simulink model "Model_pmsmdynamic"  (R2019b)
settings: Solver=ode4  StartTime=0.0  StopTime=2  RelTol=1e-3
InitFcn:
  | parameter
values from neighbouring files (symbols this model uses):
  b = 0.001    [parameter.m]
  f = 0.162    [parameter.m]
  j = 0.1    [parameter.m]
  kiid = 350    [parameter.m]
  kiiq = 350    [parameter.m]
  kis = 0.1    [parameter.m]
  kpid = 1.07    [parameter.m]
  kpiq = 1.07    [parameter.m]
  kps = 10    [parameter.m]
  Ld = 0.000538    [parameter.m]
  Lq = 0.000824    [parameter.m]
  p = 3    [parameter.m]
  rs = 0.0065    [parameter.m]
libraries: simulink x3
settings Model: ModifiedByFormat=Muhammad  Creator=Muhammad  LastModifiedBy=Muhammad
settings SolverCC: ZeroCrossAlgorithm=Adaptive
settings DataIOCC: ReturnWorkspaceOutputs=off
settings DebuggingCC: MaxConsecutiveZCsMsg=none  ArithmeticOperatorsInVariantConditions=warning
settings SFSimCC: SimUseLocalCustomCode=off  CustomCodeUndefinedFunction=UseInterfaceOnly
settings RTWCC: RTWUseLocalCustomCode=off

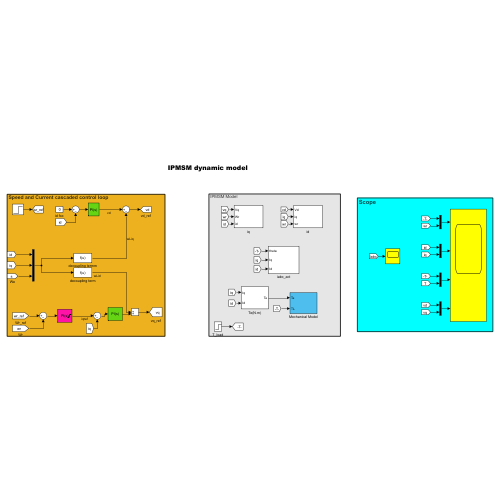
[thumbnail: Simulink's stored preview of the top-level diagram]
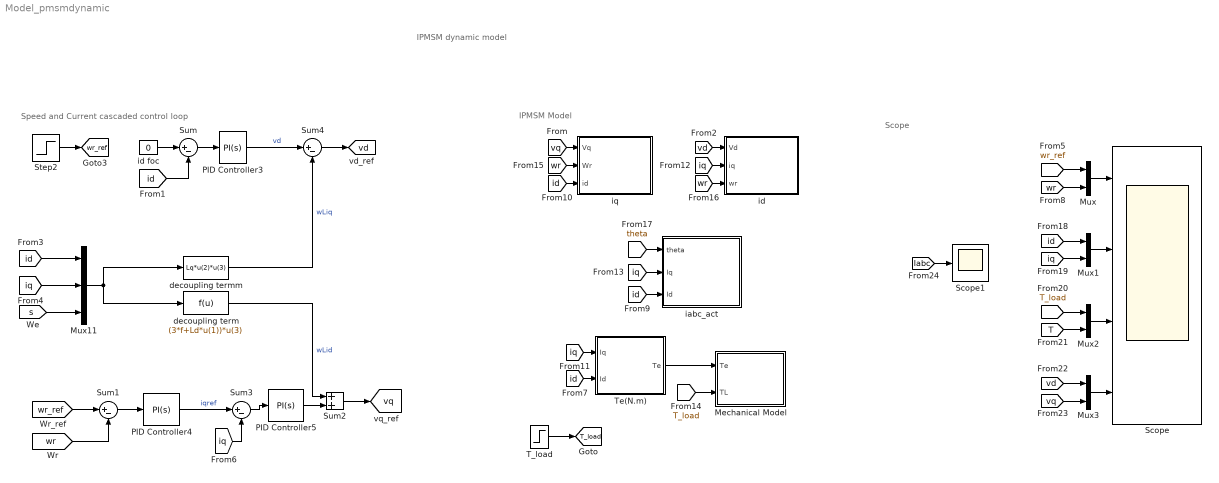
== system Model_pmsmdynamic ==
  note: Scope
  note: Speed and Current cascaded control loop
  note: IPMSM Model
  note: IPMSM dynamic model
  Mechanical Model : Subsystem
  Mux{,1..3} (4 alike) : Mux  Inputs=2
  Mux11 : Mux  Inputs=3
  PID Controller3 : simulink/Continuous/PID Controller  Controller=PI  Form=Parallel  TimeDomain=Continuous-time  SampleTime=0.0001  IntegratorMethod=Forward Euler  FilterMethod=Forward Euler  ControllerParametersSource=internal  P=kpid  I=kiid  D=0  N=100  UseFilter=on  TunerSelectOption=Transfer Function Based (PID Tuner App)  InitialConditionSource=internal  InitialConditionForIntegrator=0  InitialConditionForFilter=0  DifferentiatorICPrevScaledInput=0  ExternalReset=none  TrackingMode=off  Kt=1  LimitOutput=off  UpperSaturationLimit=800  LowerSaturationLimit=-800  LinearizeAsGain=on  AntiWindupMode=none  Kb=1  POutMin=[]  POutMax=[]  IOutMin=[]  IOutMax=[]  DOutMin=[]  DOutMax=[]  NOutMin=[]  NOutMax=[]  SumOutMin=[]  SumOutMax=[]  SaturationOutMin=[]  SaturationOutMax=[]  PParamMin=[]  PParamMax=[]  IParamMin=[]  IParamMax=[]  DParamMin=[]  DParamMax=[]  NParamMin=[]  NParamMax=[]  KbParamMin=[]  KbParamMax=[]  KtParamMin=[]  KtParamMax=[]  KbOutMin=[]  KbOutMax=[]  KtOutMin=[]  KtOutMax=[]  IntegratorOutMin=[]  IntegratorOutMax=[]  FilterOutMin=[]  FilterOutMax=[]  SumI1OutMin=[]  SumI1OutMax=[]  SumI2OutMin=[]  SumI2OutMax=[]  SumI3OutMin=[]  SumI3OutMax=[]  SumI4OutMin=[]  SumI4OutMax=[]  SumDOutMin=[]  SumDOutMax=[]  DifferentiatorOutMin=[]  DifferentiatorOutMax=[]  FilterDiffOutCoefMin=[]  FilterDiffOutCoefMax=[]  ReciprocalOutMin=[]  ReciprocalOutMax=[]  SumDenOutMin=[]  SumDenOutMax=[]  SumNumOutMin=[]  SumNumOutMax=[]  DivideOutMin=[]  DivideOutMax=[]  IntegratorContinuousStateAttributes=''  IntegratorStateMustResolveToSignalObject=off  IntegratorRTWStateStorageClass=Auto  FilterContinuousStateAttributes=''  FilterStateMustResolveToSignalObject=off  FilterRTWStateStorageClass=Auto  ParallelPVariant=InternalParameters  IdealPVariant=Disabled  IVariant=InternalParameters  DVariant=Disabled  IntegratorVariant=Continuous  SatVariant=Disabled  AWVariant=Passthrough  PCopyVariant=Disabled  TRVariant=Disabled  FdbkBlocksVariant=Forward  IdealPFdbkVariant=Disabled  SatFdbkVariant=Disabled  DerivativeFilterVariant=Disabled  NVariant=Disabled  NCopyVariant=Disabled_SignalSpec  FilterICVariant=Disabled  IntegratorICVariant=InternalICs  ExternalResetVariant=Disabled  TRSumVariant=Passthrough  SumFdbkVariant=Disabled  SumVariant=Sum_PI
  PID Controller4 : simulink/Continuous/PID Controller  Controller=PI  Form=Parallel  TimeDomain=Continuous-time  SampleTime=0.0001  IntegratorMethod=Forward Euler  FilterMethod=Forward Euler  ControllerParametersSource=internal  P=kps  I=kis  D=0  N=100  UseFilter=on  TunerSelectOption=Transfer Function Based (PID Tuner App)  InitialConditionSource=internal  InitialConditionForIntegrator=0  InitialConditionForFilter=0  DifferentiatorICPrevScaledInput=0  ExternalReset=none  TrackingMode=off  Kt=1  LimitOutput=on  UpperSaturationLimit=145  LowerSaturationLimit=-145  LinearizeAsGain=on  AntiWindupMode=none  Kb=1  POutMin=[]  POutMax=[]  IOutMin=[]  IOutMax=[]  DOutMin=[]  DOutMax=[]  NOutMin=[]  NOutMax=[]  SumOutMin=[]  SumOutMax=[]  SaturationOutMin=[]  SaturationOutMax=[]  PParamMin=[]  PParamMax=[]  IParamMin=[]  IParamMax=[]  DParamMin=[]  DParamMax=[]  NParamMin=[]  NParamMax=[]  KbParamMin=[]  KbParamMax=[]  KtParamMin=[]  KtParamMax=[]  KbOutMin=[]  KbOutMax=[]  KtOutMin=[]  KtOutMax=[]  IntegratorOutMin=[]  IntegratorOutMax=[]  FilterOutMin=[]  FilterOutMax=[]  SumI1OutMin=[]  SumI1OutMax=[]  SumI2OutMin=[]  SumI2OutMax=[]  SumI3OutMin=[]  SumI3OutMax=[]  SumI4OutMin=[]  SumI4OutMax=[]  SumDOutMin=[]  SumDOutMax=[]  DifferentiatorOutMin=[]  DifferentiatorOutMax=[]  FilterDiffOutCoefMin=[]  FilterDiffOutCoefMax=[]  ReciprocalOutMin=[]  ReciprocalOutMax=[]  SumDenOutMin=[]  SumDenOutMax=[]  SumNumOutMin=[]  SumNumOutMax=[]  DivideOutMin=[]  DivideOutMax=[]  IntegratorContinuousStateAttributes=''  IntegratorStateMustResolveToSignalObject=off  IntegratorRTWStateStorageClass=Auto  FilterContinuousStateAttributes=''  FilterStateMustResolveToSignalObject=off  FilterRTWStateStorageClass=Auto  ParallelPVariant=InternalParameters  IdealPVariant=Disabled  IVariant=InternalParameters  DVariant=Disabled  IntegratorVariant=Continuous  SatVariant=Enabled  AWVariant=Passthrough  PCopyVariant=Disabled  TRVariant=Disabled  FdbkBlocksVariant=Forward  IdealPFdbkVariant=Disabled  SatFdbkVariant=Disabled  DerivativeFilterVariant=Disabled  NVariant=Disabled  NCopyVariant=Disabled_SignalSpec  FilterICVariant=Disabled  IntegratorICVariant=InternalICs  ExternalResetVariant=Disabled  TRSumVariant=Passthrough  SumFdbkVariant=Disabled  SumVariant=Sum_PI
  PID Controller5 : simulink/Continuous/PID Controller  Controller=PI  Form=Parallel  TimeDomain=Continuous-time  SampleTime=0.0001  IntegratorMethod=Forward Euler  FilterMethod=Forward Euler  ControllerParametersSource=internal  P=kpiq  I=kiiq  D=0  N=100  UseFilter=on  TunerSelectOption=Transfer Function Based (PID Tuner App)  InitialConditionSource=internal  InitialConditionForIntegrator=0  InitialConditionForFilter=0  DifferentiatorICPrevScaledInput=0  ExternalReset=none  TrackingMode=off  Kt=1  LimitOutput=off  UpperSaturationLimit=800  LowerSaturationLimit=-800  LinearizeAsGain=on  AntiWindupMode=none  Kb=1  POutMin=[]  POutMax=[]  IOutMin=[]  IOutMax=[]  DOutMin=[]  DOutMax=[]  NOutMin=[]  NOutMax=[]  SumOutMin=[]  SumOutMax=[]  SaturationOutMin=[]  SaturationOutMax=[]  PParamMin=[]  PParamMax=[]  IParamMin=[]  IParamMax=[]  DParamMin=[]  DParamMax=[]  NParamMin=[]  NParamMax=[]  KbParamMin=[]  KbParamMax=[]  KtParamMin=[]  KtParamMax=[]  KbOutMin=[]  KbOutMax=[]  KtOutMin=[]  KtOutMax=[]  IntegratorOutMin=[]  IntegratorOutMax=[]  FilterOutMin=[]  FilterOutMax=[]  SumI1OutMin=[]  SumI1OutMax=[]  SumI2OutMin=[]  SumI2OutMax=[]  SumI3OutMin=[]  SumI3OutMax=[]  SumI4OutMin=[]  SumI4OutMax=[]  SumDOutMin=[]  SumDOutMax=[]  DifferentiatorOutMin=[]  DifferentiatorOutMax=[]  FilterDiffOutCoefMin=[]  FilterDiffOutCoefMax=[]  ReciprocalOutMin=[]  ReciprocalOutMax=[]  SumDenOutMin=[]  SumDenOutMax=[]  SumNumOutMin=[]  SumNumOutMax=[]  DivideOutMin=[]  DivideOutMax=[]  IntegratorContinuousStateAttributes=''  IntegratorStateMustResolveToSignalObject=off  IntegratorRTWStateStorageClass=Auto  FilterContinuousStateAttributes=''  FilterStateMustResolveToSignalObject=off  FilterRTWStateStorageClass=Auto  ParallelPVariant=InternalParameters  IdealPVariant=Disabled  IVariant=InternalParameters  DVariant=Disabled  IntegratorVariant=Continuous  SatVariant=Disabled  AWVariant=Passthrough  PCopyVariant=Disabled  TRVariant=Disabled  FdbkBlocksVariant=Forward  IdealPFdbkVariant=Disabled  SatFdbkVariant=Disabled  DerivativeFilterVariant=Disabled  NVariant=Disabled  NCopyVariant=Disabled_SignalSpec  FilterICVariant=Disabled  IntegratorICVariant=InternalICs  ExternalResetVariant=Disabled  TRSumVariant=Passthrough  SumFdbkVariant=Disabled  SumVariant=Sum_PI
  Scope : Scope  NumInputPorts=4
  Scope1 : Scope
  Step2 : Step  Time=0.5  Before=600  After=600  SampleTime=1e-6
  Sum{,1,3..4} (4 alike) : Sum  Inputs=|+-
  Sum2 : Sum  Inputs=|++
  T_load : Step  Before=6  After=14  SampleTime=1e-6
  Te(N.m) : Subsystem
  decoupling term : Fcn  Expr=(3*f+Ld*u(1))*u(3)
  decoupling termm : Fcn  Expr=Lq*u(2)*u(3)
  iabc_act : Subsystem
  id : Subsystem
  id foc : Constant  Value=0
  iq : Subsystem
  tag scope: T_load=global, vd=global, vq=global, wr_ref=global
  wires:
  Sum4/1 -> [vd]
  PID Controller3/1 -> Sum4/1  "vd"
  Sum2/1 -> [vq]
  PID Controller5/1 -> Sum2/2
  [s] -> Mux11/3
  Mux11/1 -> decoupling term/1, decoupling termm/1
  [id] -> Mux11/1
  [iq] -> Mux11/2
  decoupling termm/1 -> Sum4/2  "wLiq"
  Sum3/1 -> PID Controller5/1
  [iq] -> Sum3/2
  Sum/1 -> PID Controller3/1
  [wr] -> Sum1/2
  [id] -> Sum/2
  Sum1/1 -> PID Controller4/1
  id foc/1 -> Sum/1
  [vq] -> iq/1(Vq)
  [vd] -> id/1(Vd)
  Te(N.m)/1(Te) -> Mechanical Model/1(Te)
  [id] -> Te(N.m)/2(Id)
  [id] -> iabc_act/3(Id)
  [id] -> iq/3(id)
  [iq] -> Te(N.m)/1(Iq)
  [iq] -> id/2(iq)
  [iq] -> iabc_act/2(Iq)
  [wr] -> iq/2(Wr)
  [wr] -> id/3(wr)
  [theta] -> iabc_act/1(theta)
  T_load/1 -> [T_load]
  [T_load] -> Mechanical Model/2(TL)
  Step2/1 -> [wr_ref]
  [wr_ref] -> Sum1/1
  [wr_ref] -> Mux/1
  [wr] -> Mux/2
  [iq] -> Mux1/2
  [id] -> Mux1/1
  [T_load] -> Mux2/1
  [T] -> Mux2/2
  [vq] -> Mux3/2
  [vd] -> Mux3/1
  Mux/1 -> Scope/1
  Mux1/1 -> Scope/2
  Mux2/1 -> Scope/3
  Mux3/1 -> Scope/4
  [Iabc] -> Scope1/1
  decoupling term/1 -> Sum2/1  "wLid"
  PID Controller4/1 -> Sum3/1  "iqref"

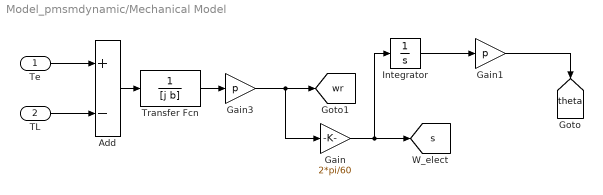
== system Model_pmsmdynamic/Mechanical Model ==
  Te : Inport
  TL : Inport  Port=2
  Add : Sum  Inputs=+-
  Gain : Gain  Gain=2*pi/60
  Gain1 : Gain  Gain=p
  Gain3 : Gain  Gain=p
  Integrator : Integrator
  Transfer Fcn : TransferFcn  Denominator=[j b]
  tag scope: s=global, theta=global, wr=global
  wires:
  TL/1 -> Add/2
  Te/1 -> Add/1
  Add/1 -> Transfer Fcn/1
  Transfer Fcn/1 -> Gain3/1
  Gain/1 -> [s], Integrator/1
  Integrator/1 -> Gain1/1
  Gain1/1 -> [theta]
  Gain3/1 -> Gain/1, [wr]

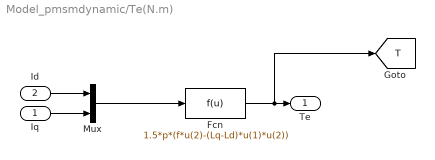
== system Model_pmsmdynamic/Te(N.m) ==
  Iq : Inport
  Id : Inport  Port=2
  Fcn : Fcn  Expr=1.5*p*(f*u(2)-(Lq-Ld)*u(1)*u(2))
  Mux : Mux  Inputs=2
  Te : Outport  VectorParamsAs1DForOutWhenUnconnected=off
  tag scope: T=global
  wires:
  Fcn/1 -> [T], Te/1
  Iq/1 -> Mux/2
  Mux/1 -> Fcn/1
  Id/1 -> Mux/1

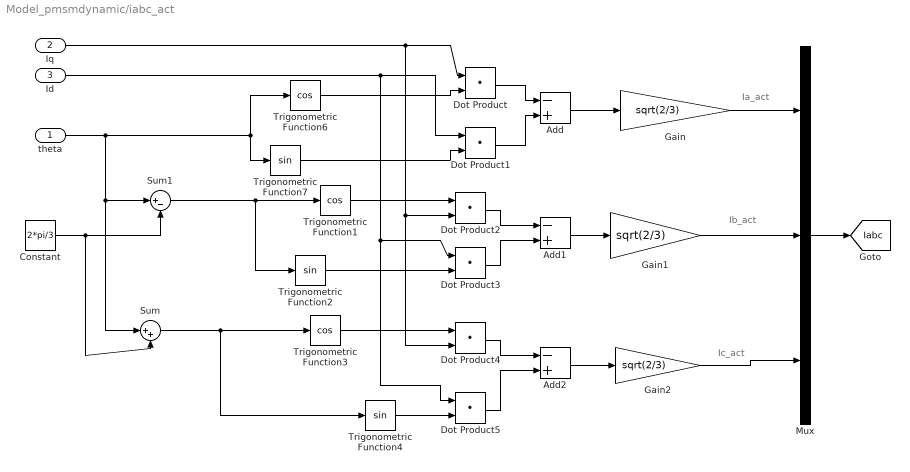
== system Model_pmsmdynamic/iabc_act ==
  note: Ia_act
  note: Ib_act
  note: Ic_act
  theta : Inport
  Iq : Inport  Port=2
  Id : Inport  Port=3
  Add : Sum  Inputs=-+
  Add1 : Sum  Inputs=-+
  Add2 : Sum  Inputs=-+
  Constant : Constant  Value=2*pi/3
  Dot Product{,1..5} (6 alike) : DotProduct  InputSameDT=on  OutDataTypeStr=Inherit: Inherit via internal rule
  Gain : Gain  Gain=sqrt(2/3)
  Gain1 : Gain  Gain=sqrt(2/3)
  Gain2 : Gain  Gain=sqrt(2/3)
  Mux : Mux  Inputs=3
  Sum : Sum  Inputs=|++
  Sum1 : Sum  Inputs=|+-
  Trigonometric Function1 : Trigonometry  Operator=cos
  Trigonometric Function2 : Trigonometry
  Trigonometric Function3 : Trigonometry  Operator=cos
  Trigonometric Function4 : Trigonometry
  Trigonometric Function6 : Trigonometry  Operator=cos
  Trigonometric Function7 : Trigonometry
  tag scope: Iabc=global
  wires:
  theta/1 -> Sum1/1, Sum/1, Trigonometric Function6/1, Trigonometric Function7/1
  Sum1/1 -> Trigonometric Function1/1, Trigonometric Function2/1
  Constant/1 -> Sum/2, Sum1/2
  Add/1 -> Gain/1
  Dot Product1/1 -> Add/2
  Dot Product/1 -> Add/1
  Trigonometric Function6/1 -> Dot Product/2
  Iq/1 -> Dot Product/1, Dot Product2/2, Dot Product4/2
  Trigonometric Function7/1 -> Dot Product1/2
  Id/1 -> Dot Product1/1, Dot Product3/1, Dot Product5/1
  Add1/1 -> Gain1/1
  Dot Product2/1 -> Add1/1
  Dot Product3/1 -> Add1/2
  Trigonometric Function1/1 -> Dot Product2/1
  Trigonometric Function2/1 -> Dot Product3/2
  Add2/1 -> Gain2/1
  Dot Product4/1 -> Add2/1
  Dot Product5/1 -> Add2/2
  Sum/1 -> Trigonometric Function3/1, Trigonometric Function4/1
  Trigonometric Function3/1 -> Dot Product4/1
  Trigonometric Function4/1 -> Dot Product5/2
  Gain/1 -> Mux/1
  Gain1/1 -> Mux/2
  Gain2/1 -> Mux/3
  Mux/1 -> [Iabc]

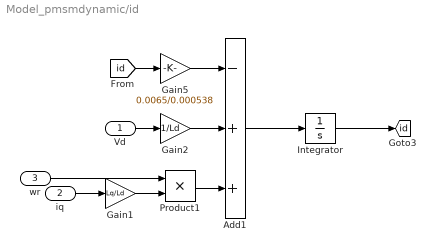
== system Model_pmsmdynamic/id ==
  Vd : Inport
  iq : Inport  Port=2
  wr : Inport  Port=3
  Add1 : Sum  Inputs=-++
  Gain1 : Gain  Gain=Lq/Ld
  Gain2 : Gain  Gain=1/Ld
  Gain5 : Gain  Gain=0.0065/0.000538
  Integrator : Integrator
  Product1 : Product  RndMeth=Zero
  tag scope: id=global
  wires:
  Integrator/1 -> [id]
  Product1/1 -> Add1/3
  wr/1 -> Product1/1
  iq/1 -> Gain1/1
  Gain1/1 -> Product1/2
  Vd/1 -> Gain2/1
  Gain5/1 -> Add1/1
  Gain2/1 -> Add1/2
  Add1/1 -> Integrator/1
  [id] -> Gain5/1

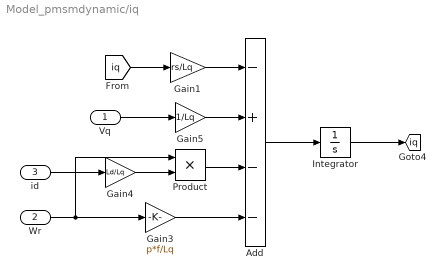
== system Model_pmsmdynamic/iq ==
  Vq : Inport
  Wr : Inport  Port=2
  id : Inport  Port=3
  Add : Sum  Inputs=-+--
  Gain1 : Gain  Gain=rs/Lq
  Gain3 : Gain  Gain=p*f/Lq
  Gain4 : Gain  Gain=Ld/Lq
  Gain5 : Gain  Gain=1/Lq
  Integrator : Integrator
  Product : Product  RndMeth=Zero
  tag scope: iq=global
  wires:
  Integrator/1 -> [iq]
  Product/1 -> Add/3
  Wr/1 -> Product/1, Gain3/1
  Gain3/1 -> Add/4
  Gain1/1 -> Add/1
  Vq/1 -> Gain5/1
  Gain4/1 -> Product/2
  id/1 -> Gain4/1
  Gain5/1 -> Add/2
  Add/1 -> Integrator/1
  [iq] -> Gain1/1
